simulink model "jointSpacePDControl"  (R2021b)
settings: Solver=VariableStepAuto  StartTime=0.0  StopTime=3  RelTol=1e-3
undefined symbols (not defined in the file): Kd, Kp, qd
settings Model: Creator=fabio  LastModifiedBy=buse

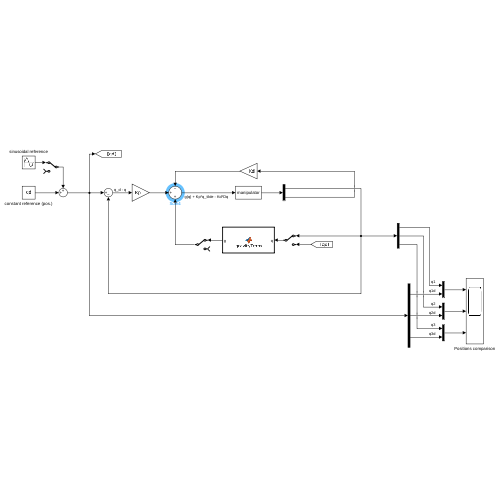
[thumbnail: Simulink's stored preview of the top-level diagram]
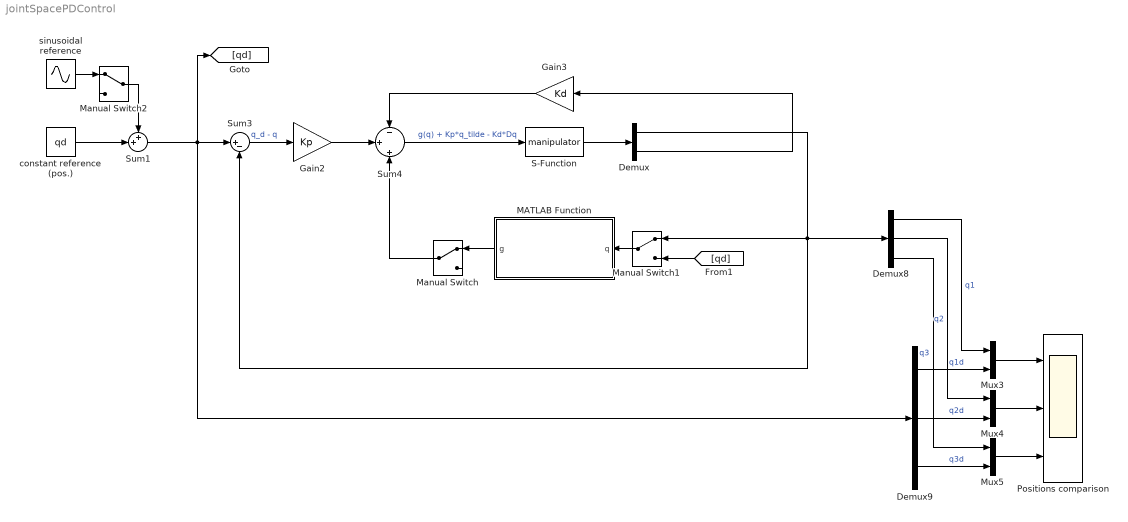
== system jointSpacePDControl ==
  Demux : Demux  Outputs=2
  Demux8 : Demux  Outputs=3
  Demux9 : Demux  Outputs=3
  Gain2 : Gain  Gain=Kp
  Gain3 : Gain  Gain=Kd
  MATLAB Function : MATLAB Function  TreatAsAtomicUnit=on
  Manual Switch : ManualSwitch
  Manual Switch1 : ManualSwitch
  Manual Switch2 : ManualSwitch
  Mux3 : Mux  Inputs=2
  Mux4 : Mux  Inputs=2
  Mux5 : Mux  Inputs=2
  Positions comparison : Scope  NumInputPorts=3
  S-Function : S-Function  FunctionName=manipulator  Parameters=robot  SFunctionDeploymentMode=off  EnableBusSupport=off
  Sum1 : Sum  Inputs=++|
  Sum3 : Sum  Inputs=|+-
  Sum4 : Sum  Inputs=-|+|+
  constant reference (pos.) : Constant  Value=qd
  sinusoidal reference : Sin  Amplitude=0.1  Frequency=2*pi  SampleTime=0
  wires:
  Demux9/2 -> Mux4/2  "q2d"
  Mux4/1 -> Positions comparison/2
  Mux3/1 -> Positions comparison/1
  Demux9/3 -> Mux5/2  "q3d"
  Sum3/1 -> Gain2/1  "q_d - q"
  Demux9/1 -> Mux3/2  "q1d"
  Demux8/2 -> Mux4/1  "q2"
  Demux8/3 -> Mux5/1  "q3"
  S-Function/1 -> Demux/1
  Demux8/1 -> Mux3/1  "q1"
  Gain2/1 -> Sum4/2
  Mux5/1 -> Positions comparison/3
  Demux/2 -> Gain3/1
  Demux/1 -> Demux8/1, Sum3/2, Manual Switch1/1
  constant reference (pos.)/1 -> Sum1/2
  sinusoidal reference/1 -> Manual Switch2/1
  Manual Switch2/1 -> Sum1/1
  Sum1/1 -> Demux9/1, [qd], Sum3/1
  Manual Switch1/1 -> MATLAB Function/1(q)
  [qd] -> Manual Switch1/2
  MATLAB Function/1(g) -> Manual Switch/1
  Manual Switch/1 -> Sum4/3
  Sum4/1 -> S-Function/1  "g(q) + Kp*q_tilde - Kd*Dq"
  Gain3/1 -> Sum4/1

== matlab function jointSpacePDControl/MATLAB Function ==
  data: q input; g output
function g = gravityTerm(q) 
    g = [             0
             0
0.9621*cos(q(3))];
end
